simulink model "pokus07_video"  (R2023a)
settings: Solver=VariableStepAuto  StartTime=0.0  StopTime=10.0  RelTol=1e-3
undefined symbols (not defined in the file): c
libraries: Miscellaneous x840, Memory_Blocks_Lib x251, Decoders_Lib x10, simulink_extras x10, Counters_Lib x4, Bit_Multiplexers_Lib x1, Byte_Multiplexers_Lib x1
(part 5 of 5)

== system pokus07_video/Character_Table/Char_N ==
  Byte_2 : Constant  Value=c.char_7x7(2, :, c.N)  OutDataTypeStr=uint8
  Byte_3 : Constant  Value=c.char_7x7(3, :, c.N)  OutDataTypeStr=uint8
  Byte_4 : Constant  Value=c.char_7x7(4, :, c.N)  OutDataTypeStr=uint8
  Byte_5 : Constant  Value=c.char_7x7(5, :, c.N)  OutDataTypeStr=uint8
  Byte_6 : Constant  Value=c.char_7x7(6, :, c.N)  OutDataTypeStr=uint8
  Byte_7 : Constant  Value=c.char_7x7(7, :, c.N)  OutDataTypeStr=uint8
  Byte_8 : Constant  Value=c.char_7x7(8, :, c.N)  OutDataTypeStr=uint8
  Byte_9 : Constant  Value=c.char_7x7(1, :, c.N)  OutDataTypeStr=uint8
  Row_7(1B) : Outport
  Row_6(1B) : Outport  Port=2
  Row_5(1B) : Outport  Port=3
  Row_4(1B) : Outport  Port=4
  Row_3(1B) : Outport  Port=5
  Row_2(1B) : Outport  Port=6
  Row_1(1B) : Outport  Port=7
  Row_0(1B) : Outport  Port=8
  wires:
  Byte_3/1 -> Row_5(1B)/1
  Byte_9/1 -> Row_7(1B)/1
  Byte_7/1 -> Row_1(1B)/1
  Byte_4/1 -> Row_4(1B)/1
  Byte_8/1 -> Row_0(1B)/1
  Byte_2/1 -> Row_6(1B)/1
  Byte_5/1 -> Row_3(1B)/1
  Byte_6/1 -> Row_2(1B)/1

== system pokus07_video/Character_Table/Char_O ==
  Byte_2 : Constant  Value=c.char_7x7(2, :, c.O)  OutDataTypeStr=uint8
  Byte_3 : Constant  Value=c.char_7x7(3, :, c.O)  OutDataTypeStr=uint8
  Byte_4 : Constant  Value=c.char_7x7(4, :, c.O)  OutDataTypeStr=uint8
  Byte_5 : Constant  Value=c.char_7x7(5, :, c.O)  OutDataTypeStr=uint8
  Byte_6 : Constant  Value=c.char_7x7(6, :, c.O)  OutDataTypeStr=uint8
  Byte_7 : Constant  Value=c.char_7x7(7, :, c.O)  OutDataTypeStr=uint8
  Byte_8 : Constant  Value=c.char_7x7(8, :, c.O)  OutDataTypeStr=uint8
  Byte_9 : Constant  Value=c.char_7x7(1, :, c.O)  OutDataTypeStr=uint8
  Row_7(1B) : Outport
  Row_6(1B) : Outport  Port=2
  Row_5(1B) : Outport  Port=3
  Row_4(1B) : Outport  Port=4
  Row_3(1B) : Outport  Port=5
  Row_2(1B) : Outport  Port=6
  Row_1(1B) : Outport  Port=7
  Row_0(1B) : Outport  Port=8
  wires:
  Byte_3/1 -> Row_5(1B)/1
  Byte_9/1 -> Row_7(1B)/1
  Byte_7/1 -> Row_1(1B)/1
  Byte_4/1 -> Row_4(1B)/1
  Byte_8/1 -> Row_0(1B)/1
  Byte_2/1 -> Row_6(1B)/1
  Byte_5/1 -> Row_3(1B)/1
  Byte_6/1 -> Row_2(1B)/1

== system pokus07_video/Character_Table/Char_P ==
  Byte_2 : Constant  Value=c.char_7x7(2, :, c.P)  OutDataTypeStr=uint8
  Byte_3 : Constant  Value=c.char_7x7(3, :, c.P)  OutDataTypeStr=uint8
  Byte_4 : Constant  Value=c.char_7x7(4, :, c.P)  OutDataTypeStr=uint8
  Byte_5 : Constant  Value=c.char_7x7(5, :, c.P)  OutDataTypeStr=uint8
  Byte_6 : Constant  Value=c.char_7x7(6, :, c.P)  OutDataTypeStr=uint8
  Byte_7 : Constant  Value=c.char_7x7(7, :, c.P)  OutDataTypeStr=uint8
  Byte_8 : Constant  Value=c.char_7x7(8, :, c.P)  OutDataTypeStr=uint8
  Byte_9 : Constant  Value=c.char_7x7(1, :, c.P)  OutDataTypeStr=uint8
  Row_7(1B) : Outport
  Row_6(1B) : Outport  Port=2
  Row_5(1B) : Outport  Port=3
  Row_4(1B) : Outport  Port=4
  Row_3(1B) : Outport  Port=5
  Row_2(1B) : Outport  Port=6
  Row_1(1B) : Outport  Port=7
  Row_0(1B) : Outport  Port=8
  wires:
  Byte_3/1 -> Row_5(1B)/1
  Byte_9/1 -> Row_7(1B)/1
  Byte_7/1 -> Row_1(1B)/1
  Byte_4/1 -> Row_4(1B)/1
  Byte_8/1 -> Row_0(1B)/1
  Byte_2/1 -> Row_6(1B)/1
  Byte_5/1 -> Row_3(1B)/1
  Byte_6/1 -> Row_2(1B)/1

== system pokus07_video/Character_Table/Char_PERCENT ==
  Byte_2 : Constant  Value=c.char_7x7(2, :, c.PERCENT)  OutDataTypeStr=uint8
  Byte_3 : Constant  Value=c.char_7x7(3, :, c.PERCENT)  OutDataTypeStr=uint8
  Byte_4 : Constant  Value=c.char_7x7(4, :, c.PERCENT)  OutDataTypeStr=uint8
  Byte_5 : Constant  Value=c.char_7x7(5, :, c.PERCENT)  OutDataTypeStr=uint8
  Byte_6 : Constant  Value=c.char_7x7(6, :, c.PERCENT)  OutDataTypeStr=uint8
  Byte_7 : Constant  Value=c.char_7x7(7, :, c.PERCENT)  OutDataTypeStr=uint8
  Byte_8 : Constant  Value=c.char_7x7(8, :, c.PERCENT)  OutDataTypeStr=uint8
  Byte_9 : Constant  Value=c.char_7x7(1, :, c.PERCENT)  OutDataTypeStr=uint8
  Row_7(1B) : Outport
  Row_6(1B) : Outport  Port=2
  Row_5(1B) : Outport  Port=3
  Row_4(1B) : Outport  Port=4
  Row_3(1B) : Outport  Port=5
  Row_2(1B) : Outport  Port=6
  Row_1(1B) : Outport  Port=7
  Row_0(1B) : Outport  Port=8
  wires:
  Byte_3/1 -> Row_5(1B)/1
  Byte_9/1 -> Row_7(1B)/1
  Byte_7/1 -> Row_1(1B)/1
  Byte_4/1 -> Row_4(1B)/1
  Byte_8/1 -> Row_0(1B)/1
  Byte_2/1 -> Row_6(1B)/1
  Byte_5/1 -> Row_3(1B)/1
  Byte_6/1 -> Row_2(1B)/1

== system pokus07_video/Character_Table/Char_PLUS ==
  Byte_2 : Constant  Value=c.char_7x7(2, :, c.PLUS)  OutDataTypeStr=uint8
  Byte_3 : Constant  Value=c.char_7x7(3, :, c.PLUS)  OutDataTypeStr=uint8
  Byte_4 : Constant  Value=c.char_7x7(4, :, c.PLUS)  OutDataTypeStr=uint8
  Byte_5 : Constant  Value=c.char_7x7(5, :, c.PLUS)  OutDataTypeStr=uint8
  Byte_6 : Constant  Value=c.char_7x7(6, :, c.PLUS)  OutDataTypeStr=uint8
  Byte_7 : Constant  Value=c.char_7x7(7, :, c.PLUS)  OutDataTypeStr=uint8
  Byte_8 : Constant  Value=c.char_7x7(8, :, c.PLUS)  OutDataTypeStr=uint8
  Byte_9 : Constant  Value=c.char_7x7(1, :, c.PLUS)  OutDataTypeStr=uint8
  Row_7(1B) : Outport
  Row_6(1B) : Outport  Port=2
  Row_5(1B) : Outport  Port=3
  Row_4(1B) : Outport  Port=4
  Row_3(1B) : Outport  Port=5
  Row_2(1B) : Outport  Port=6
  Row_1(1B) : Outport  Port=7
  Row_0(1B) : Outport  Port=8
  wires:
  Byte_3/1 -> Row_5(1B)/1
  Byte_9/1 -> Row_7(1B)/1
  Byte_7/1 -> Row_1(1B)/1
  Byte_4/1 -> Row_4(1B)/1
  Byte_8/1 -> Row_0(1B)/1
  Byte_2/1 -> Row_6(1B)/1
  Byte_5/1 -> Row_3(1B)/1
  Byte_6/1 -> Row_2(1B)/1

== system pokus07_video/Character_Table/Char_Q ==
  Byte_2 : Constant  Value=c.char_7x7(2, :, c.Q)  OutDataTypeStr=uint8
  Byte_3 : Constant  Value=c.char_7x7(3, :, c.Q)  OutDataTypeStr=uint8
  Byte_4 : Constant  Value=c.char_7x7(4, :, c.Q)  OutDataTypeStr=uint8
  Byte_5 : Constant  Value=c.char_7x7(5, :, c.Q)  OutDataTypeStr=uint8
  Byte_6 : Constant  Value=c.char_7x7(6, :, c.Q)  OutDataTypeStr=uint8
  Byte_7 : Constant  Value=c.char_7x7(7, :, c.Q)  OutDataTypeStr=uint8
  Byte_8 : Constant  Value=c.char_7x7(8, :, c.Q)  OutDataTypeStr=uint8
  Byte_9 : Constant  Value=c.char_7x7(1, :, c.Q)  OutDataTypeStr=uint8
  Row_7(1B) : Outport
  Row_6(1B) : Outport  Port=2
  Row_5(1B) : Outport  Port=3
  Row_4(1B) : Outport  Port=4
  Row_3(1B) : Outport  Port=5
  Row_2(1B) : Outport  Port=6
  Row_1(1B) : Outport  Port=7
  Row_0(1B) : Outport  Port=8
  wires:
  Byte_3/1 -> Row_5(1B)/1
  Byte_9/1 -> Row_7(1B)/1
  Byte_7/1 -> Row_1(1B)/1
  Byte_4/1 -> Row_4(1B)/1
  Byte_8/1 -> Row_0(1B)/1
  Byte_2/1 -> Row_6(1B)/1
  Byte_5/1 -> Row_3(1B)/1
  Byte_6/1 -> Row_2(1B)/1

== system pokus07_video/Character_Table/Char_QUESTION_MARK ==
  Byte_2 : Constant  Value=c.char_7x7(2, :, c.QUESTION_MARK)  OutDataTypeStr=uint8
  Byte_3 : Constant  Value=c.char_7x7(3, :, c.QUESTION_MARK)  OutDataTypeStr=uint8
  Byte_4 : Constant  Value=c.char_7x7(4, :, c.QUESTION_MARK)  OutDataTypeStr=uint8
  Byte_5 : Constant  Value=c.char_7x7(5, :, c.QUESTION_MARK)  OutDataTypeStr=uint8
  Byte_6 : Constant  Value=c.char_7x7(6, :, c.QUESTION_MARK)  OutDataTypeStr=uint8
  Byte_7 : Constant  Value=c.char_7x7(7, :, c.QUESTION_MARK)  OutDataTypeStr=uint8
  Byte_8 : Constant  Value=c.char_7x7(8, :, c.QUESTION_MARK)  OutDataTypeStr=uint8
  Byte_9 : Constant  Value=c.char_7x7(1, :, c.QUESTION_MARK)  OutDataTypeStr=uint8
  Row_7(1B) : Outport
  Row_6(1B) : Outport  Port=2
  Row_5(1B) : Outport  Port=3
  Row_4(1B) : Outport  Port=4
  Row_3(1B) : Outport  Port=5
  Row_2(1B) : Outport  Port=6
  Row_1(1B) : Outport  Port=7
  Row_0(1B) : Outport  Port=8
  wires:
  Byte_3/1 -> Row_5(1B)/1
  Byte_9/1 -> Row_7(1B)/1
  Byte_7/1 -> Row_1(1B)/1
  Byte_4/1 -> Row_4(1B)/1
  Byte_8/1 -> Row_0(1B)/1
  Byte_2/1 -> Row_6(1B)/1
  Byte_5/1 -> Row_3(1B)/1
  Byte_6/1 -> Row_2(1B)/1

== system pokus07_video/Character_Table/Char_R ==
  Byte_2 : Constant  Value=c.char_7x7(2, :, c.R)  OutDataTypeStr=uint8
  Byte_3 : Constant  Value=c.char_7x7(3, :, c.R)  OutDataTypeStr=uint8
  Byte_4 : Constant  Value=c.char_7x7(4, :, c.R)  OutDataTypeStr=uint8
  Byte_5 : Constant  Value=c.char_7x7(5, :, c.R)  OutDataTypeStr=uint8
  Byte_6 : Constant  Value=c.char_7x7(6, :, c.R)  OutDataTypeStr=uint8
  Byte_7 : Constant  Value=c.char_7x7(7, :, c.R)  OutDataTypeStr=uint8
  Byte_8 : Constant  Value=c.char_7x7(8, :, c.R)  OutDataTypeStr=uint8
  Byte_9 : Constant  Value=c.char_7x7(1, :, c.R)  OutDataTypeStr=uint8
  Row_7(1B) : Outport
  Row_6(1B) : Outport  Port=2
  Row_5(1B) : Outport  Port=3
  Row_4(1B) : Outport  Port=4
  Row_3(1B) : Outport  Port=5
  Row_2(1B) : Outport  Port=6
  Row_1(1B) : Outport  Port=7
  Row_0(1B) : Outport  Port=8
  wires:
  Byte_3/1 -> Row_5(1B)/1
  Byte_9/1 -> Row_7(1B)/1
  Byte_7/1 -> Row_1(1B)/1
  Byte_4/1 -> Row_4(1B)/1
  Byte_8/1 -> Row_0(1B)/1
  Byte_2/1 -> Row_6(1B)/1
  Byte_5/1 -> Row_3(1B)/1
  Byte_6/1 -> Row_2(1B)/1

== system pokus07_video/Character_Table/Char_S ==
  Byte_2 : Constant  Value=c.char_7x7(2, :, c.S)  OutDataTypeStr=uint8
  Byte_3 : Constant  Value=c.char_7x7(3, :, c.S)  OutDataTypeStr=uint8
  Byte_4 : Constant  Value=c.char_7x7(4, :, c.S)  OutDataTypeStr=uint8
  Byte_5 : Constant  Value=c.char_7x7(5, :, c.S)  OutDataTypeStr=uint8
  Byte_6 : Constant  Value=c.char_7x7(6, :, c.S)  OutDataTypeStr=uint8
  Byte_7 : Constant  Value=c.char_7x7(7, :, c.S)  OutDataTypeStr=uint8
  Byte_8 : Constant  Value=c.char_7x7(8, :, c.S)  OutDataTypeStr=uint8
  Byte_9 : Constant  Value=c.char_7x7(1, :, c.S)  OutDataTypeStr=uint8
  Row_7(1B) : Outport
  Row_6(1B) : Outport  Port=2
  Row_5(1B) : Outport  Port=3
  Row_4(1B) : Outport  Port=4
  Row_3(1B) : Outport  Port=5
  Row_2(1B) : Outport  Port=6
  Row_1(1B) : Outport  Port=7
  Row_0(1B) : Outport  Port=8
  wires:
  Byte_3/1 -> Row_5(1B)/1
  Byte_9/1 -> Row_7(1B)/1
  Byte_7/1 -> Row_1(1B)/1
  Byte_4/1 -> Row_4(1B)/1
  Byte_8/1 -> Row_0(1B)/1
  Byte_2/1 -> Row_6(1B)/1
  Byte_5/1 -> Row_3(1B)/1
  Byte_6/1 -> Row_2(1B)/1

== system pokus07_video/Character_Table/Char_SEMICOLON ==
  Byte_2 : Constant  Value=c.char_7x7(2, :, c.SEMICOLON)  OutDataTypeStr=uint8
  Byte_3 : Constant  Value=c.char_7x7(3, :, c.SEMICOLON)  OutDataTypeStr=uint8
  Byte_4 : Constant  Value=c.char_7x7(4, :, c.SEMICOLON)  OutDataTypeStr=uint8
  Byte_5 : Constant  Value=c.char_7x7(5, :, c.SEMICOLON)  OutDataTypeStr=uint8
  Byte_6 : Constant  Value=c.char_7x7(6, :, c.SEMICOLON)  OutDataTypeStr=uint8
  Byte_7 : Constant  Value=c.char_7x7(7, :, c.SEMICOLON)  OutDataTypeStr=uint8
  Byte_8 : Constant  Value=c.char_7x7(8, :, c.SEMICOLON)  OutDataTypeStr=uint8
  Byte_9 : Constant  Value=c.char_7x7(1, :, c.SEMICOLON)  OutDataTypeStr=uint8
  Row_7(1B) : Outport
  Row_6(1B) : Outport  Port=2
  Row_5(1B) : Outport  Port=3
  Row_4(1B) : Outport  Port=4
  Row_3(1B) : Outport  Port=5
  Row_2(1B) : Outport  Port=6
  Row_1(1B) : Outport  Port=7
  Row_0(1B) : Outport  Port=8
  wires:
  Byte_3/1 -> Row_5(1B)/1
  Byte_9/1 -> Row_7(1B)/1
  Byte_7/1 -> Row_1(1B)/1
  Byte_4/1 -> Row_4(1B)/1
  Byte_8/1 -> Row_0(1B)/1
  Byte_2/1 -> Row_6(1B)/1
  Byte_5/1 -> Row_3(1B)/1
  Byte_6/1 -> Row_2(1B)/1

== system pokus07_video/Character_Table/Char_SLASH ==
  Byte_2 : Constant  Value=c.char_7x7(2, :, c.SLASH)  OutDataTypeStr=uint8
  Byte_3 : Constant  Value=c.char_7x7(3, :, c.SLASH)  OutDataTypeStr=uint8
  Byte_4 : Constant  Value=c.char_7x7(4, :, c.SLASH)  OutDataTypeStr=uint8
  Byte_5 : Constant  Value=c.char_7x7(5, :, c.SLASH)  OutDataTypeStr=uint8
  Byte_6 : Constant  Value=c.char_7x7(6, :, c.SLASH)  OutDataTypeStr=uint8
  Byte_7 : Constant  Value=c.char_7x7(7, :, c.SLASH)  OutDataTypeStr=uint8
  Byte_8 : Constant  Value=c.char_7x7(8, :, c.SLASH)  OutDataTypeStr=uint8
  Byte_9 : Constant  Value=c.char_7x7(1, :, c.SLASH)  OutDataTypeStr=uint8
  Row_7(1B) : Outport
  Row_6(1B) : Outport  Port=2
  Row_5(1B) : Outport  Port=3
  Row_4(1B) : Outport  Port=4
  Row_3(1B) : Outport  Port=5
  Row_2(1B) : Outport  Port=6
  Row_1(1B) : Outport  Port=7
  Row_0(1B) : Outport  Port=8
  wires:
  Byte_3/1 -> Row_5(1B)/1
  Byte_9/1 -> Row_7(1B)/1
  Byte_7/1 -> Row_1(1B)/1
  Byte_4/1 -> Row_4(1B)/1
  Byte_8/1 -> Row_0(1B)/1
  Byte_2/1 -> Row_6(1B)/1
  Byte_5/1 -> Row_3(1B)/1
  Byte_6/1 -> Row_2(1B)/1

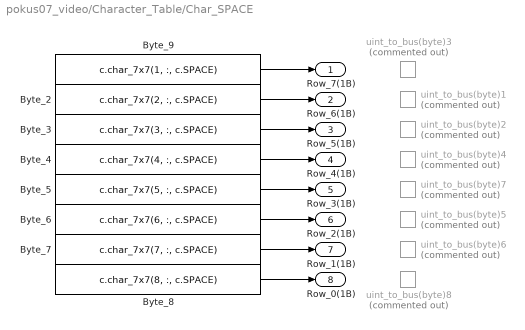
== system pokus07_video/Character_Table/Char_SPACE ==
  Byte_2 : Constant  Value=c.char_7x7(2, :, c.SPACE)  OutDataTypeStr=uint8
  Byte_3 : Constant  Value=c.char_7x7(3, :, c.SPACE)  OutDataTypeStr=uint8
  Byte_4 : Constant  Value=c.char_7x7(4, :, c.SPACE)  OutDataTypeStr=uint8
  Byte_5 : Constant  Value=c.char_7x7(5, :, c.SPACE)  OutDataTypeStr=uint8
  Byte_6 : Constant  Value=c.char_7x7(6, :, c.SPACE)  OutDataTypeStr=uint8
  Byte_7 : Constant  Value=c.char_7x7(7, :, c.SPACE)  OutDataTypeStr=uint8
  Byte_8 : Constant  Value=c.char_7x7(8, :, c.SPACE)  OutDataTypeStr=uint8
  Byte_9 : Constant  Value=c.char_7x7(1, :, c.SPACE)  OutDataTypeStr=uint8
  uint_to_bus(byte){1..8} (8 alike) : Miscellaneous/uint_to_bus(byte)  Commented=on  SystemSampleTime=-1  VariantActivationTime=update diagram  Latency=0  AutoFrameSizeCalculation=off
  Row_7(1B) : Outport
  Row_6(1B) : Outport  Port=2
  Row_5(1B) : Outport  Port=3
  Row_4(1B) : Outport  Port=4
  Row_3(1B) : Outport  Port=5
  Row_2(1B) : Outport  Port=6
  Row_1(1B) : Outport  Port=7
  Row_0(1B) : Outport  Port=8
  wires:
  Byte_3/1 -> Row_5(1B)/1
  Byte_5/1 -> Row_3(1B)/1
  Byte_8/1 -> Row_0(1B)/1
  Byte_7/1 -> Row_1(1B)/1
  Byte_4/1 -> Row_4(1B)/1
  Byte_6/1 -> Row_2(1B)/1
  Byte_9/1 -> Row_7(1B)/1
  Byte_2/1 -> Row_6(1B)/1

== system pokus07_video/Character_Table/Char_T ==
  Byte_2 : Constant  Value=c.char_7x7(2, :, c.T)  OutDataTypeStr=uint8
  Byte_3 : Constant  Value=c.char_7x7(3, :, c.T)  OutDataTypeStr=uint8
  Byte_4 : Constant  Value=c.char_7x7(4, :, c.T)  OutDataTypeStr=uint8
  Byte_5 : Constant  Value=c.char_7x7(5, :, c.T)  OutDataTypeStr=uint8
  Byte_6 : Constant  Value=c.char_7x7(6, :, c.T)  OutDataTypeStr=uint8
  Byte_7 : Constant  Value=c.char_7x7(7, :, c.T)  OutDataTypeStr=uint8
  Byte_8 : Constant  Value=c.char_7x7(8, :, c.T)  OutDataTypeStr=uint8
  Byte_9 : Constant  Value=c.char_7x7(1, :, c.T)  OutDataTypeStr=uint8
  Row_7(1B) : Outport
  Row_6(1B) : Outport  Port=2
  Row_5(1B) : Outport  Port=3
  Row_4(1B) : Outport  Port=4
  Row_3(1B) : Outport  Port=5
  Row_2(1B) : Outport  Port=6
  Row_1(1B) : Outport  Port=7
  Row_0(1B) : Outport  Port=8
  wires:
  Byte_3/1 -> Row_5(1B)/1
  Byte_9/1 -> Row_7(1B)/1
  Byte_7/1 -> Row_1(1B)/1
  Byte_4/1 -> Row_4(1B)/1
  Byte_8/1 -> Row_0(1B)/1
  Byte_2/1 -> Row_6(1B)/1
  Byte_5/1 -> Row_3(1B)/1
  Byte_6/1 -> Row_2(1B)/1

== system pokus07_video/Character_Table/Char_U ==
  Byte_2 : Constant  Value=c.char_7x7(2, :, c.U)  OutDataTypeStr=uint8
  Byte_3 : Constant  Value=c.char_7x7(3, :, c.U)  OutDataTypeStr=uint8
  Byte_4 : Constant  Value=c.char_7x7(4, :, c.U)  OutDataTypeStr=uint8
  Byte_5 : Constant  Value=c.char_7x7(5, :, c.U)  OutDataTypeStr=uint8
  Byte_6 : Constant  Value=c.char_7x7(6, :, c.U)  OutDataTypeStr=uint8
  Byte_7 : Constant  Value=c.char_7x7(7, :, c.U)  OutDataTypeStr=uint8
  Byte_8 : Constant  Value=c.char_7x7(8, :, c.U)  OutDataTypeStr=uint8
  Byte_9 : Constant  Value=c.char_7x7(1, :, c.U)  OutDataTypeStr=uint8
  Row_7(1B) : Outport
  Row_6(1B) : Outport  Port=2
  Row_5(1B) : Outport  Port=3
  Row_4(1B) : Outport  Port=4
  Row_3(1B) : Outport  Port=5
  Row_2(1B) : Outport  Port=6
  Row_1(1B) : Outport  Port=7
  Row_0(1B) : Outport  Port=8
  wires:
  Byte_3/1 -> Row_5(1B)/1
  Byte_9/1 -> Row_7(1B)/1
  Byte_7/1 -> Row_1(1B)/1
  Byte_4/1 -> Row_4(1B)/1
  Byte_8/1 -> Row_0(1B)/1
  Byte_2/1 -> Row_6(1B)/1
  Byte_5/1 -> Row_3(1B)/1
  Byte_6/1 -> Row_2(1B)/1

== system pokus07_video/Character_Table/Char_UNDERSCORE ==
  Byte_2 : Constant  Value=c.char_7x7(2, :, c.UNDERSCORE)  OutDataTypeStr=uint8
  Byte_3 : Constant  Value=c.char_7x7(3, :, c.UNDERSCORE)  OutDataTypeStr=uint8
  Byte_4 : Constant  Value=c.char_7x7(4, :, c.UNDERSCORE)  OutDataTypeStr=uint8
  Byte_5 : Constant  Value=c.char_7x7(5, :, c.UNDERSCORE)  OutDataTypeStr=uint8
  Byte_6 : Constant  Value=c.char_7x7(6, :, c.UNDERSCORE)  OutDataTypeStr=uint8
  Byte_7 : Constant  Value=c.char_7x7(7, :, c.UNDERSCORE)  OutDataTypeStr=uint8
  Byte_8 : Constant  Value=c.char_7x7(8, :, c.UNDERSCORE)  OutDataTypeStr=uint8
  Byte_9 : Constant  Value=c.char_7x7(1, :, c.UNDERSCORE)  OutDataTypeStr=uint8
  Row_7(1B) : Outport
  Row_6(1B) : Outport  Port=2
  Row_5(1B) : Outport  Port=3
  Row_4(1B) : Outport  Port=4
  Row_3(1B) : Outport  Port=5
  Row_2(1B) : Outport  Port=6
  Row_1(1B) : Outport  Port=7
  Row_0(1B) : Outport  Port=8
  wires:
  Byte_3/1 -> Row_5(1B)/1
  Byte_9/1 -> Row_7(1B)/1
  Byte_7/1 -> Row_1(1B)/1
  Byte_4/1 -> Row_4(1B)/1
  Byte_8/1 -> Row_0(1B)/1
  Byte_2/1 -> Row_6(1B)/1
  Byte_5/1 -> Row_3(1B)/1
  Byte_6/1 -> Row_2(1B)/1

== system pokus07_video/Character_Table/Char_V ==
  Byte_2 : Constant  Value=c.char_7x7(2, :, c.V)  OutDataTypeStr=uint8
  Byte_3 : Constant  Value=c.char_7x7(3, :, c.V)  OutDataTypeStr=uint8
  Byte_4 : Constant  Value=c.char_7x7(4, :, c.V)  OutDataTypeStr=uint8
  Byte_5 : Constant  Value=c.char_7x7(5, :, c.V)  OutDataTypeStr=uint8
  Byte_6 : Constant  Value=c.char_7x7(6, :, c.V)  OutDataTypeStr=uint8
  Byte_7 : Constant  Value=c.char_7x7(7, :, c.V)  OutDataTypeStr=uint8
  Byte_8 : Constant  Value=c.char_7x7(8, :, c.V)  OutDataTypeStr=uint8
  Byte_9 : Constant  Value=c.char_7x7(1, :, c.V)  OutDataTypeStr=uint8
  Row_7(1B) : Outport
  Row_6(1B) : Outport  Port=2
  Row_5(1B) : Outport  Port=3
  Row_4(1B) : Outport  Port=4
  Row_3(1B) : Outport  Port=5
  Row_2(1B) : Outport  Port=6
  Row_1(1B) : Outport  Port=7
  Row_0(1B) : Outport  Port=8
  wires:
  Byte_3/1 -> Row_5(1B)/1
  Byte_9/1 -> Row_7(1B)/1
  Byte_7/1 -> Row_1(1B)/1
  Byte_4/1 -> Row_4(1B)/1
  Byte_8/1 -> Row_0(1B)/1
  Byte_2/1 -> Row_6(1B)/1
  Byte_5/1 -> Row_3(1B)/1
  Byte_6/1 -> Row_2(1B)/1

== system pokus07_video/Character_Table/Char_W ==
  Byte_2 : Constant  Value=c.char_7x7(2, :, c.W)  OutDataTypeStr=uint8
  Byte_3 : Constant  Value=c.char_7x7(3, :, c.W)  OutDataTypeStr=uint8
  Byte_4 : Constant  Value=c.char_7x7(4, :, c.W)  OutDataTypeStr=uint8
  Byte_5 : Constant  Value=c.char_7x7(5, :, c.W)  OutDataTypeStr=uint8
  Byte_6 : Constant  Value=c.char_7x7(6, :, c.W)  OutDataTypeStr=uint8
  Byte_7 : Constant  Value=c.char_7x7(7, :, c.W)  OutDataTypeStr=uint8
  Byte_8 : Constant  Value=c.char_7x7(8, :, c.W)  OutDataTypeStr=uint8
  Byte_9 : Constant  Value=c.char_7x7(1, :, c.W)  OutDataTypeStr=uint8
  Row_7(1B) : Outport
  Row_6(1B) : Outport  Port=2
  Row_5(1B) : Outport  Port=3
  Row_4(1B) : Outport  Port=4
  Row_3(1B) : Outport  Port=5
  Row_2(1B) : Outport  Port=6
  Row_1(1B) : Outport  Port=7
  Row_0(1B) : Outport  Port=8
  wires:
  Byte_3/1 -> Row_5(1B)/1
  Byte_9/1 -> Row_7(1B)/1
  Byte_7/1 -> Row_1(1B)/1
  Byte_4/1 -> Row_4(1B)/1
  Byte_8/1 -> Row_0(1B)/1
  Byte_2/1 -> Row_6(1B)/1
  Byte_5/1 -> Row_3(1B)/1
  Byte_6/1 -> Row_2(1B)/1

== system pokus07_video/Character_Table/Char_X ==
  Byte_2 : Constant  Value=c.char_7x7(2, :, c.X)  OutDataTypeStr=uint8
  Byte_3 : Constant  Value=c.char_7x7(3, :, c.X)  OutDataTypeStr=uint8
  Byte_4 : Constant  Value=c.char_7x7(4, :, c.X)  OutDataTypeStr=uint8
  Byte_5 : Constant  Value=c.char_7x7(5, :, c.X)  OutDataTypeStr=uint8
  Byte_6 : Constant  Value=c.char_7x7(6, :, c.X)  OutDataTypeStr=uint8
  Byte_7 : Constant  Value=c.char_7x7(7, :, c.X)  OutDataTypeStr=uint8
  Byte_8 : Constant  Value=c.char_7x7(8, :, c.X)  OutDataTypeStr=uint8
  Byte_9 : Constant  Value=c.char_7x7(1, :, c.X)  OutDataTypeStr=uint8
  Row_7(1B) : Outport
  Row_6(1B) : Outport  Port=2
  Row_5(1B) : Outport  Port=3
  Row_4(1B) : Outport  Port=4
  Row_3(1B) : Outport  Port=5
  Row_2(1B) : Outport  Port=6
  Row_1(1B) : Outport  Port=7
  Row_0(1B) : Outport  Port=8
  wires:
  Byte_3/1 -> Row_5(1B)/1
  Byte_9/1 -> Row_7(1B)/1
  Byte_7/1 -> Row_1(1B)/1
  Byte_4/1 -> Row_4(1B)/1
  Byte_8/1 -> Row_0(1B)/1
  Byte_2/1 -> Row_6(1B)/1
  Byte_5/1 -> Row_3(1B)/1
  Byte_6/1 -> Row_2(1B)/1

== system pokus07_video/Character_Table/Char_Y ==
  Byte_2 : Constant  Value=c.char_7x7(2, :, c.Y)  OutDataTypeStr=uint8
  Byte_3 : Constant  Value=c.char_7x7(3, :, c.Y)  OutDataTypeStr=uint8
  Byte_4 : Constant  Value=c.char_7x7(4, :, c.Y)  OutDataTypeStr=uint8
  Byte_5 : Constant  Value=c.char_7x7(5, :, c.Y)  OutDataTypeStr=uint8
  Byte_6 : Constant  Value=c.char_7x7(6, :, c.Y)  OutDataTypeStr=uint8
  Byte_7 : Constant  Value=c.char_7x7(7, :, c.Y)  OutDataTypeStr=uint8
  Byte_8 : Constant  Value=c.char_7x7(8, :, c.Y)  OutDataTypeStr=uint8
  Byte_9 : Constant  Value=c.char_7x7(1, :, c.Y)  OutDataTypeStr=uint8
  Row_7(1B) : Outport
  Row_6(1B) : Outport  Port=2
  Row_5(1B) : Outport  Port=3
  Row_4(1B) : Outport  Port=4
  Row_3(1B) : Outport  Port=5
  Row_2(1B) : Outport  Port=6
  Row_1(1B) : Outport  Port=7
  Row_0(1B) : Outport  Port=8
  wires:
  Byte_3/1 -> Row_5(1B)/1
  Byte_9/1 -> Row_7(1B)/1
  Byte_7/1 -> Row_1(1B)/1
  Byte_4/1 -> Row_4(1B)/1
  Byte_8/1 -> Row_0(1B)/1
  Byte_2/1 -> Row_6(1B)/1
  Byte_5/1 -> Row_3(1B)/1
  Byte_6/1 -> Row_2(1B)/1

== system pokus07_video/Character_Table/Char_Z ==
  Byte_2 : Constant  Value=c.char_7x7(2, :, c.Z)  OutDataTypeStr=uint8
  Byte_3 : Constant  Value=c.char_7x7(3, :, c.Z)  OutDataTypeStr=uint8
  Byte_4 : Constant  Value=c.char_7x7(4, :, c.Z)  OutDataTypeStr=uint8
  Byte_5 : Constant  Value=c.char_7x7(5, :, c.Z)  OutDataTypeStr=uint8
  Byte_6 : Constant  Value=c.char_7x7(6, :, c.Z)  OutDataTypeStr=uint8
  Byte_7 : Constant  Value=c.char_7x7(7, :, c.Z)  OutDataTypeStr=uint8
  Byte_8 : Constant  Value=c.char_7x7(8, :, c.Z)  OutDataTypeStr=uint8
  Byte_9 : Constant  Value=c.char_7x7(1, :, c.Z)  OutDataTypeStr=uint8
  Row_7(1B) : Outport
  Row_6(1B) : Outport  Port=2
  Row_5(1B) : Outport  Port=3
  Row_4(1B) : Outport  Port=4
  Row_3(1B) : Outport  Port=5
  Row_2(1B) : Outport  Port=6
  Row_1(1B) : Outport  Port=7
  Row_0(1B) : Outport  Port=8
  wires:
  Byte_3/1 -> Row_5(1B)/1
  Byte_9/1 -> Row_7(1B)/1
  Byte_7/1 -> Row_1(1B)/1
  Byte_4/1 -> Row_4(1B)/1
  Byte_8/1 -> Row_0(1B)/1
  Byte_2/1 -> Row_6(1B)/1
  Byte_5/1 -> Row_3(1B)/1
  Byte_6/1 -> Row_2(1B)/1
